simulink model "test_ellman"  (R2017a)
settings: Solver=VariableStepAuto  StartTime=0.0  StopTime=1  RelTol=1e-3
undefined symbols (not defined in the file or in its folder): magnitude
libraries: usask_hyd_lib_simulink x2, simulink x1
settings Model: Creator=tkw954  LastModifiedBy=tkw954

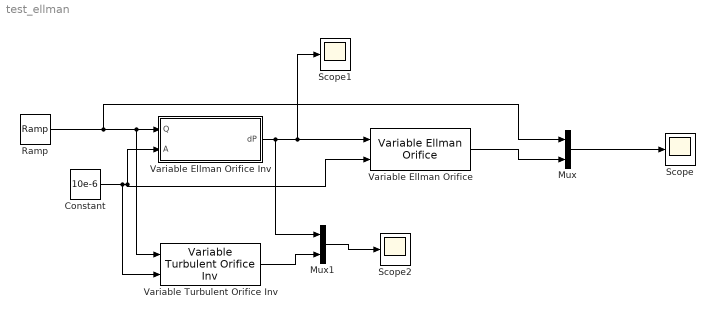
== system test_ellman ==
  Constant : Constant  Value=10e-6
  Mux : Mux  Inputs=2
  Mux1 : Mux  Inputs=2
  Ramp : simulink/Sources/Ramp  slope=3e-6  start=0  X0=0
  Scope : Scope
  Scope1 : Scope
  Scope2 : Scope
  Variable Ellman Orifice : usask_hyd_lib_simulink/Variable Ellman Orifice  rho=800  nu=30e-6  Cd=0.61  Re_cr=12  A0=1e-9
      settings: SourceProductName=USask Hydraulic Library Simulink
  Variable Ellman Orifice Inv : Subsystem  mask(Turbulent Orifice){rho=800, nu=30e-6, Cd=0.61, Re_cr=12, A0=1e-9}
      mask prompts: rho "Fluid Density (kg/m^3)"; nu "Fluid Kinematic Viscosity (m^2/s)"; Cd "Discharge Coefficient"; Re_cr "Critical Reynolds Number"; A0 "Lekage Area (m^2)"
      mask help: This block implements Ellman's two region orifice equation. This implementation calculates hydraulic diameter assuming a circular orifice.
  Variable Turbulent Orifice Inv : usask_hyd_lib_simulink/Variable Turbulent Orifice Inv  rho=800  Cd=0.61  A0=1e-9
      settings: SourceProductName=USask Hydraulic Library Simulink
  wires:
  Ramp/1 -> Mux/1, Variable Turbulent Orifice Inv/1, Variable Ellman Orifice Inv/1(Q)
  Constant/1 -> Variable Turbulent Orifice Inv/2, Variable Ellman Orifice Inv/2(A), Variable Ellman Orifice/2
  Variable Ellman Orifice/1 -> Mux/2
  Mux1/1 -> Scope2/1
  Variable Turbulent Orifice Inv/1 -> Mux1/2
  Variable Ellman Orifice Inv/1(dP) -> Mux1/1, Scope1/1, Variable Ellman Orifice/1
  Mux/1 -> Scope/1

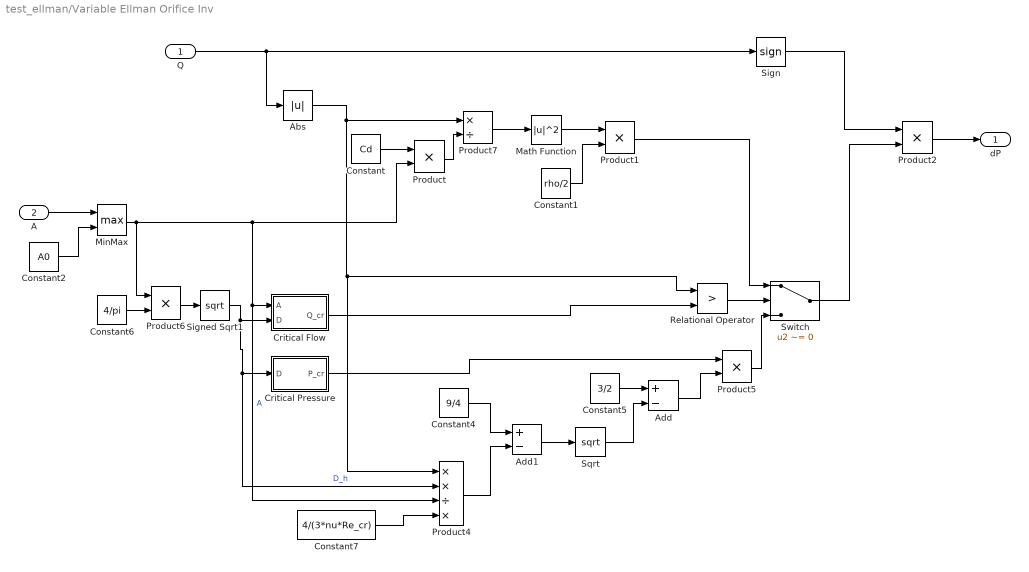
== system test_ellman/Variable Ellman Orifice Inv ==
  Q : Inport
  A : Inport  Port=2
  Abs : Abs
  Add : Sum  Inputs=+-
  Add1 : Sum  Inputs=+-
  Constant : Constant  Value=Cd
  Constant1 : Constant  Value=rho/2
  Constant2 : Constant  Value=A0
  Constant4 : Constant  Value=9/4
  Constant5 : Constant  Value=3/2
  Constant6 : Constant  Value=4/pi
  Constant7 : Constant  Value=4/(3*nu*Re_cr)
  Critical Flow : Subsystem
  Critical Pressure : Subsystem
  Math Function : Math  Operator=magnitude^2  SaturateOnIntegerOverflow=on
  MinMax : MinMax  Function=max  Inputs=2
  Product{,1..2,6} (4 alike) : Product
  Product4 : Product  Inputs=**/*
  Product5 : Product  Inputs=**
  Product7 : Product  Inputs=*/
  Relational Operator : RelationalOperator  Operator=>  OutDataTypeStr=boolean  RndMeth=Nearest
  Sign : Signum
  Signed Sqrt1 : Sqrt  SaturateOnIntegerOverflow=on
  Sqrt : Sqrt  SaturateOnIntegerOverflow=on
  Switch : Switch  Criteria=u2 ~= 0
  dP : Outport
  wires:
  Abs/1 -> Product7/1, Product4/1, Relational Operator/1
  Constant/1 -> Product/1
  Q/1 -> Sign/1, Abs/1
  Constant1/1 -> Product1/2
  A/1 -> MinMax/1
  MinMax/1 -> Product6/1, Product4/3, Critical Flow/1(A), Product/2  "A"
  Constant2/1 -> MinMax/2
  Product2/1 -> dP/1
  Sign/1 -> Product2/1
  Switch/1 -> Product2/2
  Relational Operator/1 -> Switch/2
  Product1/1 -> Switch/1
  Product5/1 -> Switch/3
  Constant5/1 -> Add/1
  Product6/1 -> Signed Sqrt1/1
  Signed Sqrt1/1 -> Critical Flow/2(D), Product4/2, Critical Pressure/1(D)  "D_h"
  Constant6/1 -> Product6/2
  Critical Flow/1(Q_cr) -> Relational Operator/2
  Product/1 -> Product7/2
  Product7/1 -> Math Function/1
  Math Function/1 -> Product1/1
  Critical Pressure/1(P_cr) -> Product5/1
  Add/1 -> Product5/2
  Sqrt/1 -> Add/2
  Add1/1 -> Sqrt/1
  Constant4/1 -> Add1/1
  Product4/1 -> Add1/2
  Constant7/1 -> Product4/4

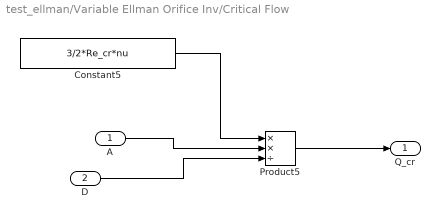
== system test_ellman/Variable Ellman Orifice Inv/Critical Flow ==
  A : Inport
  D : Inport  Port=2
  Constant5 : Constant  Value=3/2*Re_cr*nu
  Product5 : Product  Inputs=**/
  Q_cr : Outport
  wires:
  Constant5/1 -> Product5/1
  Product5/1 -> Q_cr/1
  D/1 -> Product5/3
  A/1 -> Product5/2

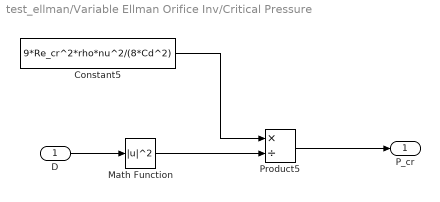
== system test_ellman/Variable Ellman Orifice Inv/Critical Pressure ==
  D : Inport
  Constant5 : Constant  Value=9*Re_cr^2*rho*nu^2/(8*Cd^2)
  Math Function : Math  Operator=magnitude^2  SaturateOnIntegerOverflow=on
  Product5 : Product  Inputs=*/
  P_cr : Outport
  wires:
  Constant5/1 -> Product5/1
  D/1 -> Math Function/1
  Product5/1 -> P_cr/1
  Math Function/1 -> Product5/2
